simulink model "nxtracer_ctrl"  (Simulink 6.4)
settings: Solver=FixedStepDiscrete  SolverMode=SingleTasking  StartTime=0  StopTime=inf  FixedStep=0.001  RelTol=1e-3
PreLoadFcn:
  | param;
libraries: ecrobot_nxt_lib x14
CloseFcn:
  | rtwprivate ssgencode ModelCloseRequest nxtcar_ctrl
settings Model: Creator=tchikama  LastModifiedBy=tchikama  ProdHWDeviceType=ARM7
settings DataIOCC: LimitDataPoints=off  SaveOutput=off  SignalLogging=off  SaveTime=off
settings OptimizationCC: InlineParams=on  InlineInvariantSignals=on  RollThreshold=2  StateBitsets=on  DataBitsets=on  UseTempVars=on  InitFltsAndDblsToZero=off  NoFixptDivByZeroProtection=on  EfficientFloat2IntCast=on  OptimizeModelRefInitCode=on  LifeSpan=1
settings DebuggingCC: ConsistencyChecking=warning  SignalInfNanChecking=warning  ReadBeforeWriteMsg=DisableAll  WriteAfterWriteMsg=DisableAll  WriteAfterReadMsg=DisableAll  AlgebraicLoopMsg=error  CheckExecutionContextPreStartOutputMsg=on  CheckExecutionContextRuntimeOutputMsg=on  SolverPrmCheckMsg=none  SingleTaskRateTransMsg=warning  TasksWithSamePriorityMsg=none  IntegerOverflowMsg=error  ParameterUnderflowMsg=warning  ParameterPrecisionLossMsg=none  UnconnectedInputMsg=error  UnconnectedOutputMsg=error  UnconnectedLineMsg=error  UniqueDataStoreMsg=error  BusObjectLabelMismatch=error  RootOutportRequireBusObject=error  ModelReferenceIOMsg=warning  ModelReferenceVersionMismatchMessage=warning  ModelReferenceIOMismatchMessage=warning
settings HardwareCC: ProdIntDivRoundTo=Zero  ProdEndianess=LittleEndian  ProdHWDeviceType=ARM7  TargetHWDeviceType=32-bit Generic
settings ModelReferenceCC: ModelReferenceNumInstancesAllowed=Single
settings RTWCC: SystemTargetFile=ert.tlc  GenCodeOnly=on  GenerateMakefile=off  TemplateMakefile=ert_default_tmf  Description=Real-Time Workshop Embedded Coder (no auto configuration)  GenerateReport=on  RTWVerbose=off  ProcessScript=ert_make_rtw_hook  IncludeHyperlinkInReport=on  LaunchReport=on  IncludeBusHierarchyInRTWFileBlockHierarchyMap=on
settings CodeAppCC: ForceParamTrailComments=on  IgnoreCustomStorageClasses=off  SFDataObjDesc=on  PrefixModelToSubsysFcnNames=off  CustomSymbolStrGlobalVar=rt$N$M  CustomSymbolStrType=$N$M  CustomSymbolStrFcn=$N$M$F  CustomSymbolStrMacro=$N$M  InsertBlockDesc=on
settings ERTTargetCC: TargetFcnLib=ansi_tfl_tmw.mat  GenFloatMathFcnCalls=GNU  IncludeMdlTerminateFcn=off  SuppressErrorStatus=on  IncludeERTFirstTime=on  SupportAbsoluteTime=off  SupportNonFinite=off  SupportComplex=off  PurelyIntegerCode=on  InlinedParameterPlacement=NonHierarchical  RootIOFormat=Structure reference  ERTCustomFileTemplate=example_file_process.tlc  InitialValueSource=Model

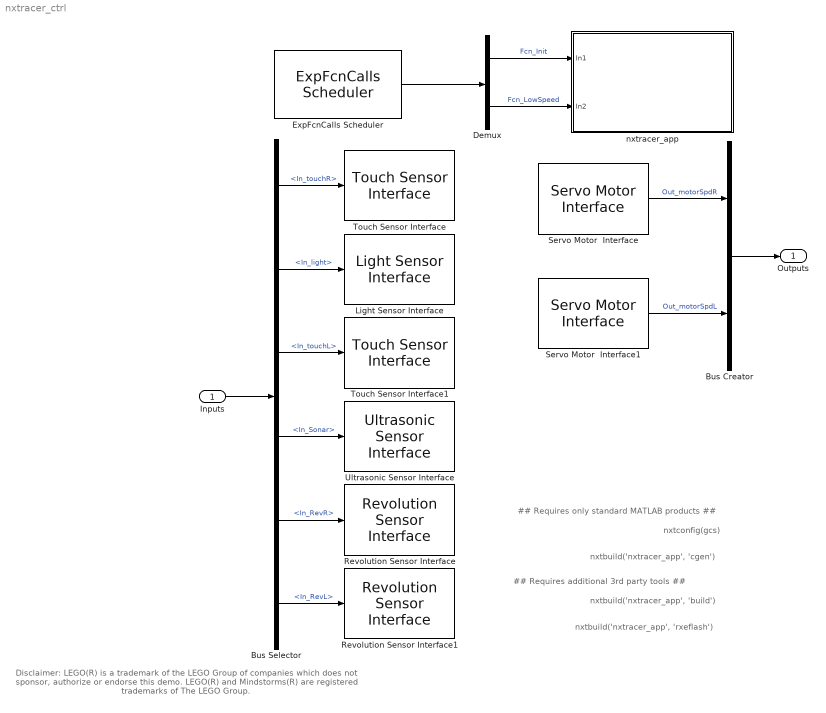
== system nxtracer_ctrl ==
  note: nxtbuild('nxtracer_app', 'cgen')
  note: nxtconfig(gcs)
  note: Disclaimer:
      | LEGO(R) is a trademark of the LEGO Group of companies which does not sponsor, authorize or endorse this demo.
      | LEGO(R) and Mindstorms(R) are registered trademarks of The LEGO Group.
  note: nxtbuild('nxtracer_app', 'build')
  note: nxtbuild('nxtracer_app', 'rxeflash')
  note: ## Requires only standard MATLAB products ##
  note: ## Requires additional 3rd party tools ##
  Inputs : Inport  UseBusObject=on
      settings: BusObject=Inputs
  Bus Creator : BusCreator  Inputs=2  UseBusObject=on
      settings: BusObject=Outputs
  Bus Selector : BusSelector  OutputSignals=In_touchR,In_light,In_touchL,In_Sonar,In_RevR,In_RevL
  Demux : Demux  Outputs=2
  ExpFcnCalls Scheduler : ecrobot_nxt_lib/ExpFcnCalls Scheduler  Priority=50  fcname='Fcn_Init', 'Fcn_LowSpeed'  fctrigger=[0 10]  ts=0.001  platform=OSEK  stacksize=[512 512]  bd_mode=Slave
  Light Sensor Interface : ecrobot_nxt_lib/Light Sensor Interface  Priority=1  SystemSampleTime=-1  ip=S4
  Revolution Sensor Interface : ecrobot_nxt_lib/Revolution Sensor Interface  Priority=3  SystemSampleTime=-1  ip=A
  Revolution Sensor Interface1 : ecrobot_nxt_lib/Revolution Sensor Interface  Priority=4  SystemSampleTime=-1  ip=B
  Servo Motor  Interface : ecrobot_nxt_lib/Servo Motor Interface  Priority=100  SystemSampleTime=-1  ip=A  mode=Brake
  Servo Motor  Interface1 : ecrobot_nxt_lib/Servo Motor Interface  Priority=101  SystemSampleTime=-1  ip=B  mode=Brake
  Touch Sensor Interface : ecrobot_nxt_lib/Touch Sensor Interface  Priority=0  SystemSampleTime=-1  ip=S2
  Touch Sensor Interface1 : ecrobot_nxt_lib/Touch Sensor Interface  Priority=2  SystemSampleTime=-1  ip=S3
  Ultrasonic Sensor Interface : ecrobot_nxt_lib/Ultrasonic Sensor Interface  SystemSampleTime=-1  ip=S1
  nxtracer_app : Subsystem
  Outputs : Outport  UseBusObject=on
      settings: BusObject=Outputs
  wires:
  Bus Selector/2 -> Light Sensor Interface/1  "<In_light>"
  Bus Selector/5 -> Revolution Sensor Interface/1  "<In_RevR>"
  Bus Selector/6 -> Revolution Sensor Interface1/1  "<In_RevL>"
  Bus Creator/1 -> Outputs/1
  Inputs/1 -> Bus Selector/1
  Bus Selector/1 -> Touch Sensor Interface/1  "<In_touchR>"
  Bus Selector/3 -> Touch Sensor Interface1/1  "<In_touchL>"
  Servo Motor  Interface/1 -> Bus Creator/1  "Out_motorSpdR"
  Servo Motor  Interface1/1 -> Bus Creator/2  "Out_motorSpdL"
  ExpFcnCalls Scheduler/1 -> Demux/1
  Demux/1 -> nxtracer_app/1(In1)  "Fcn_Init"
  Demux/2 -> nxtracer_app/2(In2)  "Fcn_LowSpeed"
  Bus Selector/4 -> Ultrasonic Sensor Interface/1  "<In_Sonar>"

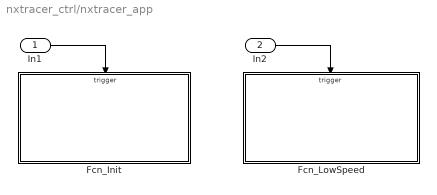
== system nxtracer_ctrl/nxtracer_app ==
  In1 : Inport
  In2 : Inport  Port=2
  Fcn_Init : Subsystem  TreatAsAtomicUnit=on
  Fcn_LowSpeed : Subsystem  TreatAsAtomicUnit=on
  wires:
  In1/1 -> Fcn_Init/Trigger
  In2/1 -> Fcn_LowSpeed/Trigger

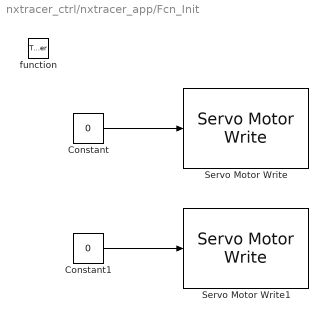
== system nxtracer_ctrl/nxtracer_app/Fcn_Init ==
  function : TriggerPort  TriggerType=function-call
  Constant : Constant  Value=0  OutDataType=sfix(16)  ConRadixGroup=Use specified scaling  OutScaling=2^0  SampleTime=inf  FramePeriod=inf
  Constant1 : Constant  Value=0  OutDataType=sfix(16)  ConRadixGroup=Use specified scaling  OutScaling=2^0  SampleTime=inf  FramePeriod=inf
  Servo Motor Write : ecrobot_nxt_lib/Servo Motor Write  SystemSampleTime=-1  ip=A
  Servo Motor Write1 : ecrobot_nxt_lib/Servo Motor Write  SystemSampleTime=-1  ip=B
  wires:
  Constant/1 -> Servo Motor Write/1
  Constant1/1 -> Servo Motor Write1/1

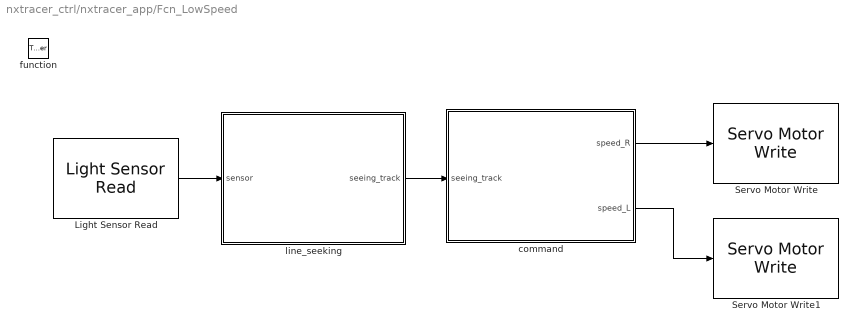
== system nxtracer_ctrl/nxtracer_app/Fcn_LowSpeed ==
  function : TriggerPort  TriggerType=function-call
  Light Sensor Read : ecrobot_nxt_lib/Light Sensor Read  SystemSampleTime=-1  ip=S4
  Servo Motor Write : ecrobot_nxt_lib/Servo Motor Write  SystemSampleTime=-1  ip=A
  Servo Motor Write1 : ecrobot_nxt_lib/Servo Motor Write  SystemSampleTime=-1  ip=B
  command : Stateflow chart
      settings: RTWSystemCode=Function  RTWFcnNameOpts=Use subsystem name
  line_seeking : Stateflow chart  TreatAsAtomicUnit=on
      settings: RTWSystemCode=Function  RTWFcnNameOpts=Use subsystem name
  wires:
  Light Sensor Read/1 -> line_seeking/1(sensor)
  line_seeking/1(seeing_track) -> command/1(seeing_track)
  command/1(speed_R) -> Servo Motor Write/1
  command/2(speed_L) -> Servo Motor Write1/1

== stateflow chart nxtracer_app/Fcn_LowSpeed/line_seeking ==
  state sensor_sees_white /
    entry: seeing_track=0;
  state sensor_sees_black /
    entry: seeing_track=1;
  state sensor_initialize/
    entry: seeing_track=0;
    (junction 11) -> sensor_initialize : {max1=mv[1];}
    sensor_initialize -> (junction 6) [order 1] : {cnt++;}
    (junction 6) -> (junction 7) [order 1] : [mv[0] > sensor]
    (junction 8) -> (junction 9) : {min1=mv[0];}
    (junction 6) -> (junction 8) [order 2]
    (junction 7) -> (junction 12) : {mv[0]=sensor;}
    (junction 9) -> (junction 11) [order 2]
    (junction 9) -> (junction 10) [order 1] : [mv[1]<sensor]
    (junction 10) -> (junction 13) : {mv[1]=sensor;}
    (junction 12) -> (junction 8)
    (junction 13) -> (junction 11)
  sensor_sees_white  -> sensor_sees_black  : [sensor>=(2*max1+min1)/3]
  sensor_sees_black  -> sensor_sees_white  : [sensor<= (max1+2*min1)/3]
  sensor_initialize -> sensor_sees_black  [order 1] : [cnt>150]
  (default) -> sensor_initialize : {mv[0]=sensor;mv[1]=sensor;}
  data: sensor input uint16; seeing_track output boolean; cnt local uint16 =0; mv local uint16 size=2; max1 local uint16; min1 local uint16
  data sensor settings: description=sensor output, maybe filtered
  data seeing_track settings: description=true if sensor is on track where track color=black on white

== stateflow chart nxtracer_app/Fcn_LowSpeed/command ==
  state Turn/
    (history)
    state Turn_Left
      entry:
      speed_R = 40;
      speed_L = -40;
      during:
      cnt1++;
    state Turn_Right
      entry:
      speed_R = -40;
      speed_L = 40;
      during:
      cnt2++;
    (default) -> Turn_Left
    Turn_Left -> Turn_Right : [(cnt1>50) && (flag ==0)]{flag=1;}
    Turn_Right -> Turn_Left : [(cnt2>50) && (flag ==0)]{flag=1;}
  state follow_line
    entry:
    speed_R = 100;
    speed_L = 100;
  Turn -> follow_line : [seeing_track==1]
      | {flag=0;
      | cnt1=0;
      | cnt2=0;}
  (default) -> follow_line
  follow_line -> Turn : [seeing_track==0]
  data: seeing_track input boolean; cnt1 local uint16; cnt2 local uint16; flag local boolean; speed_R output int8; speed_L output int8
